simulink model "InvPendulumSim"  (R2021a)
settings: Solver=VariableStepAuto  StartTime=0.0  StopTime=10.0  RelTol=1e-3
values from neighbouring files (symbols this model uses):
  A = [0 1 0 0 ... (first row only)    [Simulink.m]
  B = [0; 1/(M*l); 0; 1/M]    [Simulink.m]
undefined symbols (not defined in the file or in its folder): K
settings Model: RequirementInfo="{}  %GIDa_90b3d609_77b9_47de_8eef_c90a1886568e"  Creator=ginorospigliosi  LastModifiedBy=ginorospigliosi

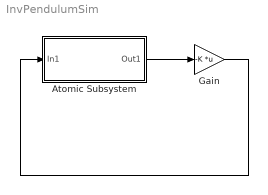
== system InvPendulumSim ==
  Atomic Subsystem : Subsystem  TreatAsAtomicUnit=on
  Gain : Gain  Gain=-K  Multiplication=Matrix(K*u)
  wires:
  Atomic Subsystem/1(Out1) -> Gain/1
  Gain/1 -> Atomic Subsystem/1(In1)

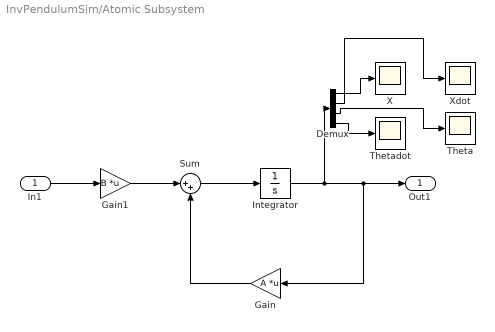
== system InvPendulumSim/Atomic Subsystem ==
  In1 : Inport
  Demux : Demux
  Gain : Gain  Gain=A  Multiplication=Matrix(K*u)
  Gain1 : Gain  Gain=B  Multiplication=Matrix(K*u)
  Integrator : Integrator  InitialCondition=[0.1; 0; 0; 0]
  Sum : Sum  Inputs=|++
  Theta : Scope
  Thetadot : Scope
  X : Scope
  Xdot : Scope
  Out1 : Outport
  wires:
  In1/1 -> Gain1/1
  Gain1/1 -> Sum/1
  Gain/1 -> Sum/2
  Integrator/1 -> Demux/1, Gain/1, Out1/1
  Sum/1 -> Integrator/1
  Demux/4 -> Thetadot/1
  Demux/3 -> Theta/1
  Demux/1 -> X/1
  Demux/2 -> Xdot/1
